simulink model "inner_mellinger_control"  (R2016a)
settings: Solver=VariableStepAuto  StartTime=0.0  StopTime=10  RelTol=1e-3
undefined symbols (not defined in the file or in its folder): inner_h, k
libraries: vrlib x2
settings Model: Creator=Daniel  LastModifiedBy=mgreiff
settings DataIOCC: LimitDataPoints=on
settings DebuggingCC: AllowSymbolicDim=off
settings ModelReferenceCC: PropagateSignalLabelsOutOfModel=off
settings GRTTargetCC: GeneratePreprocessorConditionals=Use local settings

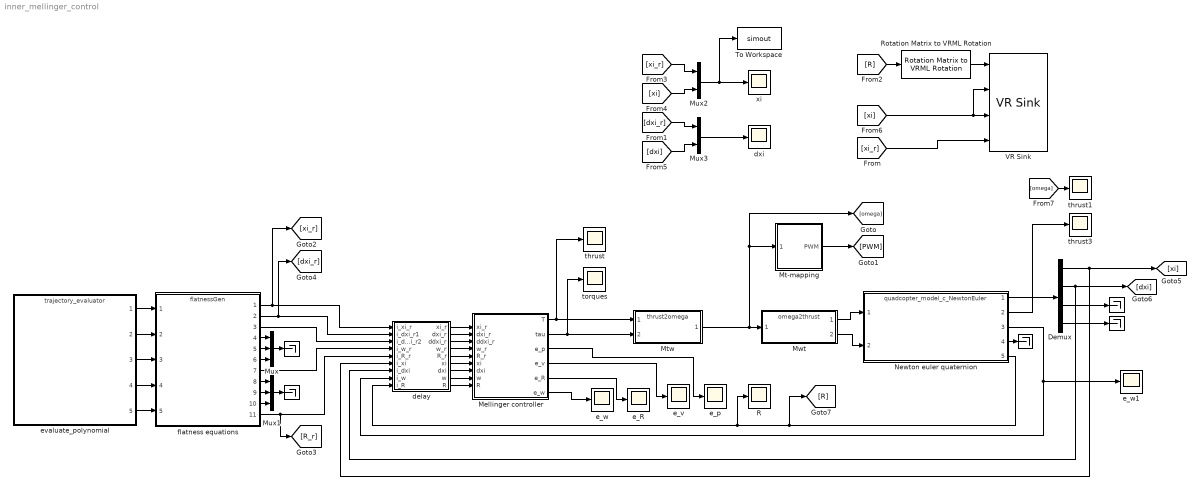
== system inner_mellinger_control ==
  " " : Terminator
  "  " : Terminator
  "     " : Terminator
  "      " : Terminator
  "       " : Terminator
  Demux : Demux  Outputs=[3,3,3,3]
  Mellinger controller : MATLAB Function  TreatAsAtomicUnit=on  SystemSampleTime=inner_h
  Mt-mapping : Subsystem
  Mtw : ModelReference  ModelNameDialog=thrust2omega.mdl  SimulationMode=Normal  ModelReferenceVersion=1.3
  Mux : Mux  Inputs=3
  Mux1 : Mux  Inputs=3
  Mux2 : Mux  Inputs=2
  Mux3 : Mux  Inputs=2
  Mwt : ModelReference  ModelNameDialog=omega2thrust.mdl  SimulationMode=Normal  ModelReferenceVersion=1.3
  Newton euler quaternion : ModelReference  ModelNameDialog=quadcopter_model_c_NewtonEuler.mdl  SimulationMode=Normal  ModelReferenceVersion=1.325
  R : Scope
  Rotation Matrix to VRML Rotation : vrlib/Utilities/Rotation Matrix to VRML Rotation  maxzero=1e-12
  To Workspace : ToWorkspace  VariableName=simout  SaveFormat=Timeseries  SampleTime=-1
  VR Sink : vrlib/VR Sink  InstantiateOnLoad=on  SampleTime=0.05  ViewEnable=on  RemoteChange=off  RemoteView=off  FieldsWritten=copter.rotation.4.1.1.double#copter.translation.3.1.1.double#vp.translation.3.1.1.double#target.translation.3.1.1.double  WorldFileName=copter_world.wrl  WorldDescription=quadcopter_world  AutoView=on  VideoDimensions=[]  AllowVariableSize=off
  delay : Subsystem
  dxi : Scope
  e_R : Scope
  e_p : Scope
  e_v : Scope
  e_w : Scope
  e_w1 : Scope
  evaluate_polynomial : ModelReference  ModelNameDialog=trajectory_evaluator.slx  SimulationMode=Normal  ModelReferenceVersion=1.106
  flatness equations : ModelReference  ModelNameDialog=flatnessGen.slx  SimulationMode=Normal  ModelReferenceVersion=1.117
  thrust : Scope
  thrust1 : Scope
  thrust3 : Scope
  torques : Scope
  xi : Scope
  wires:
  Mt-mapping/1(PWM) -> [PWM]
  Mwt/1 -> Newton euler quaternion/1
  Mwt/2 -> Newton euler quaternion/2
  evaluate_polynomial/1 -> flatness equations/1
  evaluate_polynomial/2 -> flatness equations/2
  evaluate_polynomial/3 -> flatness equations/3
  evaluate_polynomial/4 -> flatness equations/4
  evaluate_polynomial/5 -> flatness equations/5
  Mellinger controller/2(tau) -> torques/1, Mtw/2
  flatness equations/1 -> delay/1(i_xi_r), [xi_r]
  Newton euler quaternion/1 -> Demux/1
  Newton euler quaternion/2 -> thrust3/1
  Demux/2 -> delay/7(i_dxi), [dxi]
  Demux/1 -> delay/6(i_xi), [xi]
  Newton euler quaternion/4 -> "     "/1
  Mux1/1 -> "  "/1
  Mux/1 -> " "/1
  flatness equations/8 -> Mux1/1
  flatness equations/9 -> Mux1/2
  flatness equations/10 -> Mux1/3
  flatness equations/4 -> Mux/1
  flatness equations/5 -> Mux/2
  flatness equations/6 -> Mux/3
  flatness equations/7 -> delay/4(i_w_r)
  flatness equations/3 -> delay/3(i_ddxi_r2)
  flatness equations/11 -> delay/5(i_R_r), [R_r]
  flatness equations/2 -> delay/2(i_dxi_r1), [dxi_r]
  Newton euler quaternion/5 -> [R], delay/9(i_R), R/1
  Rotation Matrix to VRML Rotation/1 -> VR Sink/1
  [R] -> Rotation Matrix to VRML Rotation/1
  Mux2/1 -> To Workspace/1, xi/1
  Mux3/1 -> dxi/1
  [xi_r] -> Mux2/1
  [dxi_r] -> Mux3/1
  Demux/3 -> "      "/1
  Demux/4 -> "       "/1
  [xi] -> Mux2/2
  [dxi] -> Mux3/2
  Mellinger controller/6(e_w) -> e_w/1
  Mellinger controller/5(e_R) -> e_R/1
  Mellinger controller/4(e_v) -> e_v/1
  Mellinger controller/3(e_p) -> e_p/1
  [xi] -> VR Sink/2, VR Sink/3
  [omega] -> thrust1/1
  Newton euler quaternion/3 -> e_w1/1, delay/8(i_w)
  delay/1(xi_r) -> Mellinger controller/1(xi_r)
  delay/2(dxi_r) -> Mellinger controller/2(dxi_r)
  delay/3(ddxi_r) -> Mellinger controller/3(ddxi_r)
  delay/4(w_r) -> Mellinger controller/4(w_r)
  delay/5(R_r) -> Mellinger controller/5(R_r)
  delay/6(xi) -> Mellinger controller/6(xi)
  delay/7(dxi) -> Mellinger controller/7(dxi)
  delay/8(w) -> Mellinger controller/8(w)
  delay/9(R) -> Mellinger controller/9(R)
  Mellinger controller/1(T) -> Mtw/1, thrust/1
  Mtw/1 -> Mt-mapping/1(omega), [omega], Mwt/1
  [xi_r] -> VR Sink/4

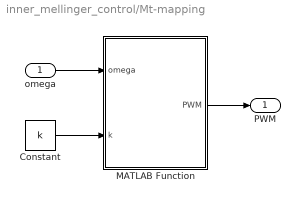
== system inner_mellinger_control/Mt-mapping ==
  omega : Inport
  Constant : Constant  Value=k
  MATLAB Function : MATLAB Function  TreatAsAtomicUnit=on
  PWM : Outport
  wires:
  MATLAB Function/1(PWM) -> PWM/1
  omega/1 -> MATLAB Function/1(omega)
  Constant/1 -> MATLAB Function/2(k)

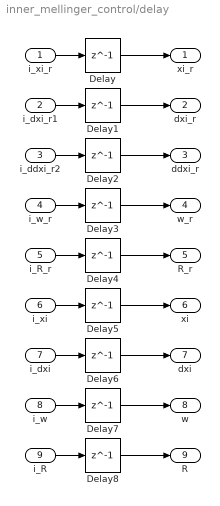
== system inner_mellinger_control/delay ==
  i_xi_r : Inport
  i_dxi_r1 : Inport  Port=2
  i_ddxi_r2 : Inport  Port=3
  i_w_r : Inport  Port=4
  i_R_r : Inport  Port=5
  i_xi : Inport  Port=6
  i_dxi : Inport  Port=7
  i_w : Inport  Port=8
  i_R : Inport  Port=9
  Delay{,1..8} (9 alike) : Delay  DelayLength=1  InitialCondition=0  SampleTime=inner_h
  xi_r : Outport
  dxi_r : Outport  Port=2
  ddxi_r : Outport  Port=3
  w_r : Outport  Port=4
  R_r : Outport  Port=5
  xi : Outport  Port=6
  dxi : Outport  Port=7
  w : Outport  Port=8
  R : Outport  Port=9
  wires:
  Delay/1 -> xi_r/1
  Delay1/1 -> dxi_r/1
  Delay2/1 -> ddxi_r/1
  Delay4/1 -> R_r/1
  Delay3/1 -> w_r/1
  Delay5/1 -> xi/1
  Delay6/1 -> dxi/1
  Delay8/1 -> R/1
  Delay7/1 -> w/1
  i_xi_r/1 -> Delay/1
  i_ddxi_r2/1 -> Delay2/1
  i_dxi_r1/1 -> Delay1/1
  i_w_r/1 -> Delay3/1
  i_R_r/1 -> Delay4/1
  i_xi/1 -> Delay5/1
  i_dxi/1 -> Delay6/1
  i_w/1 -> Delay7/1
  i_R/1 -> Delay8/1

== matlab function inner_mellinger_control/Mellinger controller ==
  data: xi_r input; dxi_r input; ddxi_r input; w_r input; R_r input; xi input; T output; tau output; dxi input; w input; R input; e_p output; e_v output; e_R output; e_w output
function [T, tau, e_p, e_v, e_R, e_w] = controller(xi_r, dxi_r, ddxi_r, w_r, R_r, xi, dxi, w, R)
%I = [0.0820; 0.0845; 0.1377];
%A=[0;0;0]
%m = 4.34;

m = 0.027;
g = 9.81;
% Functional tuning for type A
K_p = 0.2 * eye(3);
K_v = 0.025 * eye(3);
K_R = 0.1 * eye(3);
K_w = 0.001 * eye(3);

% Functional tuning for type B
K_p = 0.4 * eye(3);
K_v = 0.1* eye(3);
K_R = 0.4 * eye(3);
K_w = 0.01 * eye(3);

K_p = 0.8 * eye(3);
K_v = 0.12* eye(3);
K_R = 0.5 * eye(3);
K_w = 0.005 * eye(3);

%#codegen
zw = [0; 0; 1];
zb = R(:,3);

e_p = xi_r - xi;
e_v = dxi_r - dxi;
F_des = K_p * e_p + K_v * e_v + m * g * zw + m * ddxi_r;
T = F_des'*zb;

zb_des = F_des./ norm(F_des);
psi = 0;
yc_des = [cos(psi+pi/2); sin(psi+pi/2); 0];
xb_des = cross(yc_des, zb_des)./norm(cross(yc_des, zb_des));
yb_des = cross(zb_des, xb_des);
R_des = [xb_des, yb_des, zb_des];

Ssym = 0.5.* (R_des' * R - R' * R_des);
e_R = -[Ssym(3,2); Ssym(1,3); Ssym(2,1)]; % Vee map
e_w = (w_r - w);

%disp([norm(e_p), norm(e_v), norm(e_R), norm(e_w)])

tau = K_R * e_R + K_w * e_w;

== matlab function inner_mellinger_control/Mt-mapping/MATLAB Function ==
  data: omega input; PWM output; k input
function PWM = Mt(omega, k)
%#codegen
rotor_thrusts = k.*omega.^2;
beta1 = 0.0877;
beta2 = 0.0660;
PWM =  -beta1/(2*beta2) + sqrt((beta1/(2*beta2))^2 + rotor_thrusts/beta2);
